simulink model "exercise1"  (R2024b)
settings: Solver=VariableStepAuto  StartTime=0.0  StopTime=2  RelTol=1e-3
undefined symbols (not defined in the file): A, A_v, g, K, rho
settings Model: Creator=sadra  LastModifiedBy=sadra

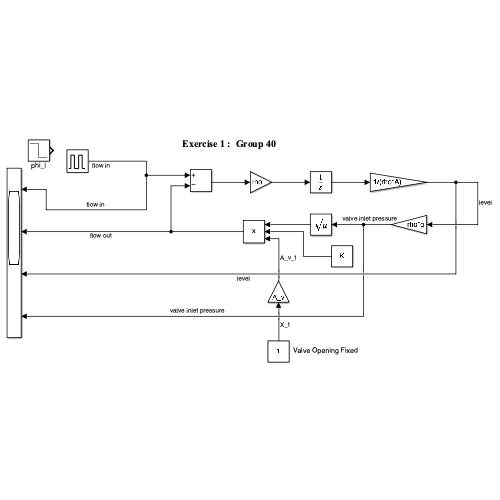
[thumbnail: Simulink's stored preview of the top-level diagram]
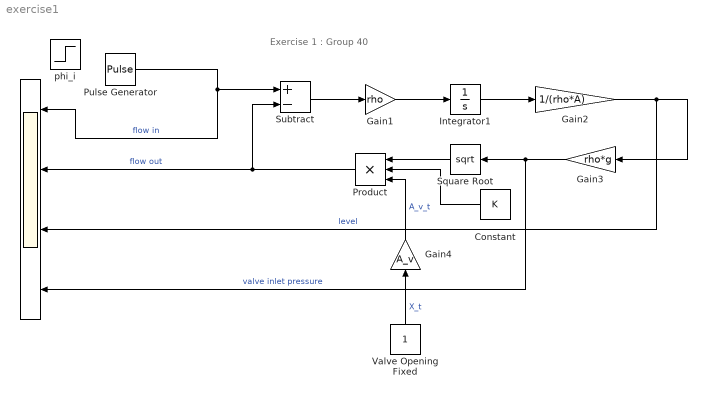
== system exercise1 ==
  note: Exercise 1 : Group 40
  " " : Scope  NumInputPorts=4
  Constant : Constant  Value=K
  Gain1 : Gain  Gain=rho
  Gain2 : Gain  Gain=1/(rho*A)
  Gain3 : Gain  Gain=rho*g
  Gain4 : Gain  Gain=A_v
  Integrator1 : Integrator
  Product : Product  Inputs=3
  Pulse Generator : DiscretePulseGenerator  PulseType=Time based  Amplitude=10  Period=1  PulseWidth=50  PhaseDelay=0.25
  Square Root : Sqrt
  Subtract : Sum  Inputs=+-
  Valve Opening Fixed : Constant
  phi_i : Step  Time=0.25  Before=10  After=5  SampleTime=0
  wires:
  Product/1 -> Subtract/2, " "/2  "flow out"
  Pulse Generator/1 -> " "/1, Subtract/1  "flow in"
  Subtract/1 -> Gain1/1
  Gain1/1 -> Integrator1/1
  Integrator1/1 -> Gain2/1
  Gain2/1 -> " "/3, Gain3/1  "level"
  Gain3/1 -> " "/4, Square Root/1  "valve inlet pressure"
  Square Root/1 -> Product/1
  Constant/1 -> Product/2
  Valve Opening Fixed/1 -> Gain4/1  "X_t"
  Gain4/1 -> Product/3  "A_v_t"
